simulink model "FullBridgeDA_DA_Converter"  (R2018a)
settings: Solver=VariableStepAuto  StartTime=0.0  StopTime=0.01  RelTol=1e-3
libraries: powerlib x14, powerlib_meascontrol x2
settings Model: Creator=ozie  LastModifiedBy=ozie

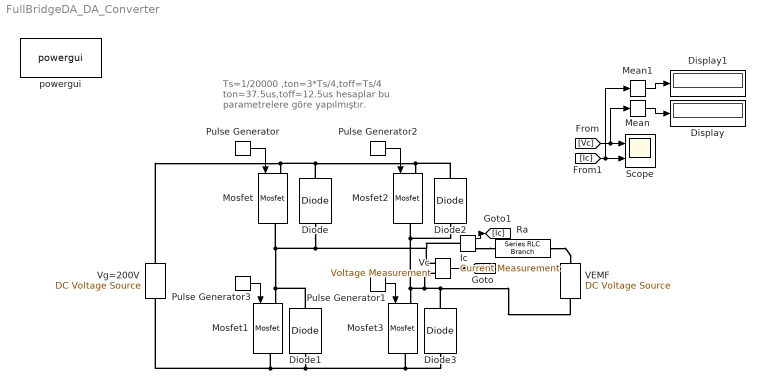
== system FullBridgeDA_DA_Converter ==
  note: Ts=1/20000 ,ton=3*Ts/4,toff=Ts/4
      |
      | ton=37.5us,toff=12.5us  hesaplar bu parametrelere göre yapılmıştır.
  Diode{,1..3} (4 alike) : powerlib/Power Electronics/Diode  Ron=0.001  Lon=0  Vf=0  IC=0  UseSnubber=0  Rs=500  Cs=250e-9  Measurements=off
  Display : Display
      settings: Format=bank
  Display1 : Display
      settings: Format=bank
  Ic : powerlib/Measurements/Current Measurement  PhasorSimulation=off  OutputType=Complex  PSBequivalent=0
  Mean : powerlib_meascontrol/Measurements/Mean  Freq=20000  Vinit=0  Ts=0
  Mean1 : powerlib_meascontrol/Measurements/Mean  Freq=20000  Vinit=0  Ts=0
  Mosfet{,1..3} (4 alike) : powerlib/Power Electronics/Mosfet  Ron=0.1  Lon=0  Rd=0.01  Vfd=0  IC=0  Rs=1e5  Cs=inf  Measurements=off
  Pulse Generator : DiscretePulseGenerator  PulseType=Time based  Period=1/20000  PulseWidth=75  PhaseDelay=12.5e-6
  Pulse Generator1 : DiscretePulseGenerator  PulseType=Time based  Period=1/20000  PulseWidth=75  PhaseDelay=12.5e-6
  Pulse Generator2 : DiscretePulseGenerator  PulseType=Time based  Period=1/20000  PulseWidth=25
  Pulse Generator3 : DiscretePulseGenerator  PulseType=Time based  Period=1/20000  PulseWidth=25
  Ra : powerlib/Elements/Series RLC Branch  LConnTagsString=__new0  RConnTagsString=__new0  BranchType=R  Resistance=2  Inductance=1e-3  SetiL0=off  InitialCurrent=0  Capacitance=1e-6  Setx0=off  InitialVoltage=0  Measurements=None
  Scope : Scope  NumInputPorts=2
  VEMF : powerlib/Electrical Sources/DC Voltage Source  Amplitude=50  Measurements=None
  Vc : powerlib/Measurements/Voltage Measurement  PhasorSimulation=off  OutputType=Complex  PSBequivalent=0
  Vg=200V : powerlib/Electrical Sources/DC Voltage Source  Amplitude=200  Measurements=None
  powergui : powerlib/powergui  Priority=1  SimulationMode=Continuous  SampleTime=50e-6  frequency=60  Iterations=50  frequencyindice=0  Pbase=100e6  ErrMax=1e-4  UnitsV=kV  UnitsW=MW  buscounter=0  FunctionMessages=off  echomessages=off  EnableUseOfTLC=off  CurrentSourceSwitches=off  DisableSnubberDevices=off  DisableRonSwitches=off  DisableVfSwitches=off  DisplayEquations=off  SolverType=Tustin/Backward Euler (TBE)  Interpol=off  ExternalGateDelay=off  methode=off  Ts=100  x0status=blocks  SPID=on  SwTol=0  HookPort=off  RestoreLinks=warning  ResistiveCurrentMeasurement=off  Frange=[0:2:500]  Ylog=off  Xlog=on  ShowGrid=off  save=off  variable=ZData  structure=0  ZoomFFT=off  StartTime=0.0  cycles=1  DisplayStyle=1  fundamental=60  FreqAxis=off  MaxFrequency=1000  frequencyindicesteady=1  RmsSteady=1  display=off
  wires:
  Pulse Generator/1 -> Mosfet/1
  Pulse Generator1/1 -> Mosfet3/1
  Pulse Generator2/1 -> Mosfet2/1
  Pulse Generator3/1 -> Mosfet1/1
  Vc/1 -> [Vc]
  [Vc] -> Mean/1, Scope/1
  Ic/1 -> [Ic]
  [Ic] -> Mean1/1, Scope/2
  Mean/1 -> Display/1
  Mean1/1 -> Display1/1
  connections:
  Diode/LConn1 -- Ic/LConn1 -- Vc/LConn1 -- Diode1/RConn1 -- Mosfet1/LConn1 -- Mosfet/RConn1
  Diode3/LConn1 -- Diode1/LConn1 -- Vg=200V/LConn1 -- Mosfet1/RConn1 -- Mosfet3/RConn1
  Diode/RConn1 -- Mosfet2/LConn1 -- Diode2/RConn1 -- Vg=200V/RConn1 -- Mosfet/LConn1
  Diode3/RConn1 -- Vc/LConn2 -- Mosfet2/RConn1 -- Diode2/LConn1 -- Mosfet3/LConn1 -- VEMF/LConn1
  Ra/RConn1 -- VEMF/RConn1
  Ic/RConn1 -- Ra/LConn1
